simulink model "model_old"  (R2020a)
settings: Solver=FixedStepDiscrete  StartTime=0.0  StopTime=inf  RelTol=1e-3
undefined symbols (not defined in the file): pause
libraries: dspvision x1, visionsources x1, simulink x1, visionanalysis x1
settings Model: Creator=thema  LastModifiedBy=thema

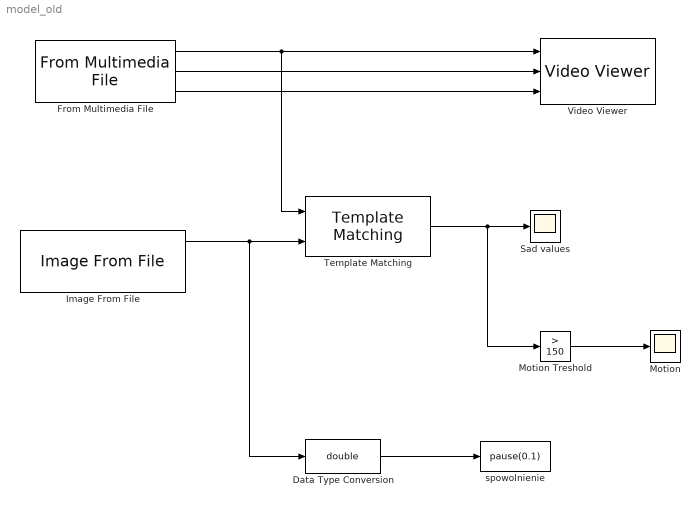
== system model_old ==
  Data Type Conversion : DataTypeConversion  OutDataTypeStr=double
  From Multimedia File : dspvision/From Multimedia File  inputFilename=motion1.avi  readRange=[1 Inf]  loop=on  numPlays=inf  outputStreams=Video only  videoDataType=uint8  audioDataType=int16  inheritSampleTime=on  userDefinedSampleTime=1/30  noAudioOutput=off  isIntensityVideo=off  fourcc=RGB  colorVideoFormat=Separate color signals  outputEOF=off  dataOrg=Column-major  audioFrameSize=1024  computeAudioFrameSize=off  outSamplingMode=Sample based
  Image From File : visionsources/Image From File  Tag=vipblks_nd  FileName=tlo0000.bmp  Ts=inf  imagePorts=Separate color signals  OutPortLabels=R|G|B  ImageDataType=Inherit from input image  sdImageDataType=uint(8)  Signed=on  WordLength=16  FractionLengthMode=User-defined  FractionLength=15
  Motion : Scope
  Motion Treshold : simulink/Logic and Bit Operations/Compare To Constant  relop=>  const=150  OutDataTypeStr=boolean
  Sad values : Scope
  Template Matching : visionanalysis/Template Matching  metric=Sum of absolute differences  output=Metric matrix  method=Exhaustive  nMetric=off  nSize=3  roi=off  roiValid=off  roundingMode=Floor  overflowMode=off  prodOutputMode=Binary point scaling  prodOutputWordLength=32  prodOutputFracLength=0  accumMode=Binary point scaling  accumWordLength=32  accumFracLength=0  outputMode=Binary point scaling  outputWordLength=32  outputFracLength=0
      settings: SourceProductBaseCode=VP
  Video Viewer : VideoViewer  imagePorts=separate color signals  FigPos=[-985.4 993.2 418.4 304]
  spowolnienie : MATLABFcn  MATLABFcn=pause(0.1)  OutputDimensions=0
  wires:
  From Multimedia File/1 -> Video Viewer/1, Template Matching/1
  From Multimedia File/2 -> Video Viewer/2
  From Multimedia File/3 -> Video Viewer/3
  Image From File/1 -> Template Matching/2, Data Type Conversion/1
  Template Matching/1 -> Motion Treshold/1, Sad values/1
  Motion Treshold/1 -> Motion/1
  Data Type Conversion/1 -> spowolnienie/1
